simulink subsystem "Reefscape_Teleop_sub"  (R2023b)
settings: Solver=VariableStepAuto  StartTime=0.0  StopTime=10.0  RelTol=1e-3
libraries: simulink x13
settings Model: Creator=ander  LastModifiedBy=ander

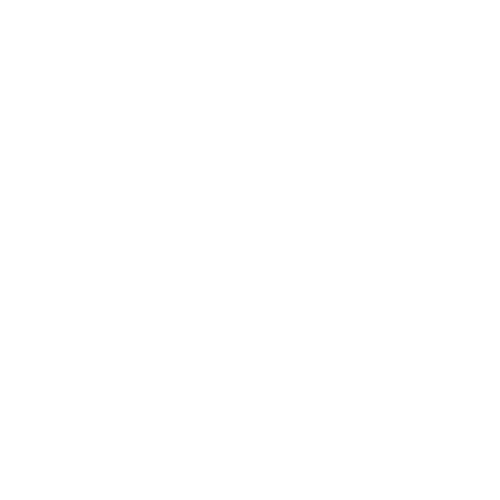
[thumbnail: Simulink's stored preview of the top-level diagram]
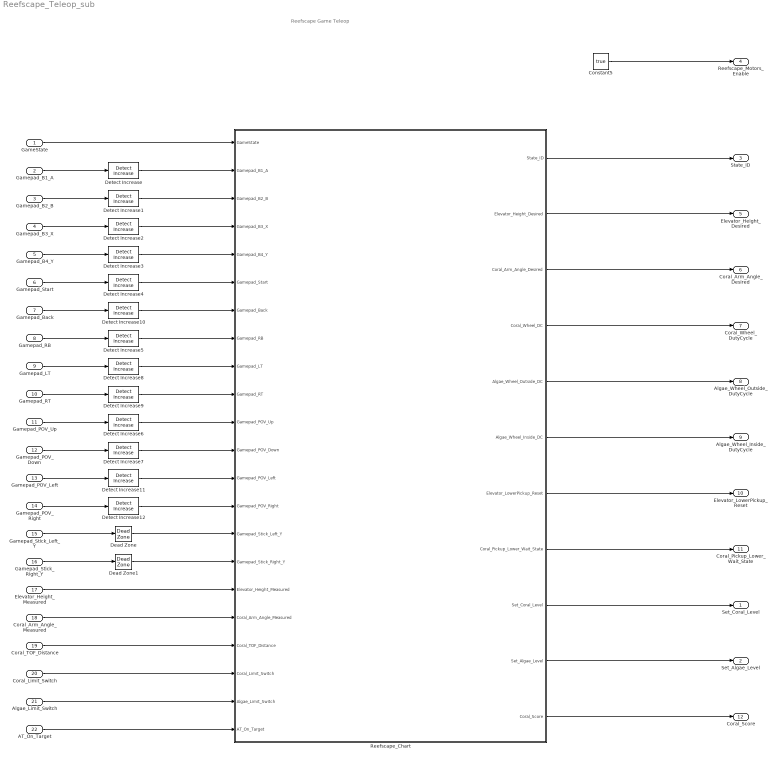
== system Reefscape_Teleop_sub ==
  note: Reefscape Game Teleop
  GameState : Inport
  Gamepad_B1_A : Inport  Port=2
  Gamepad_B2_B : Inport  Port=3
  Gamepad_B3_X : Inport  Port=4
  Gamepad_B4_Y : Inport  Port=5
  Gamepad_Start : Inport  Port=6
  Gamepad_Back : Inport  Port=7
  Gamepad_RB : Inport  Port=8
  Gamepad_LT : Inport  Port=9
  Gamepad_RT : Inport  Port=10
  Gamepad_POV_Up : Inport  Port=11
  Gamepad_POV_Down : Inport  Port=12
  Gamepad_POV_Left : Inport  Port=13
  Gamepad_POV_Right : Inport  Port=14
  Gamepad_Stick_Left_Y : Inport  Port=15
  Gamepad_Stick_Right_Y : Inport  Port=16
  Elevator_Height_Measured : Inport  Port=17
  Coral_Arm_Angle_Measured : Inport  Port=18
  Coral_TOF_Distance : Inport  Port=19
  Coral_Limit_Switch : Inport  Port=20
  Algae_Limit_Switch : Inport  Port=21
  AT_On_Target : Inport  Port=22
  Constant5 : Constant  Value=true
  Dead Zone : DeadZone  LowerValue=-0.1  UpperValue=0.1
  Dead Zone1 : DeadZone  LowerValue=-0.1  UpperValue=0.1
  Detect Increase{,1..12} (13 alike) : simulink/Logic and Bit Operations/Detect Increase  vinit=0.0  OutDataTypeStr=boolean
  Reefscape_Chart : Stateflow chart  TreatAsAtomicUnit=on
  Set_Coral_Level : Outport
  Set_Algae_Level : Outport  Port=2
  State_ID : Outport  Port=3
  Reefscape_Motors_Enable : Outport  Port=4
  Elevator_Height_Desired : Outport  Port=5
  Coral_Arm_Angle_Desired : Outport  Port=6
  Coral_Wheel_DutyCycle : Outport  Port=7
  Algae_Wheel_Outside_DutyCycle : Outport  Port=8
  Algae_Wheel_Inside_DutyCycle : Outport  Port=9
  Elevator_LowerPickup_Reset : Outport  Port=10
  Coral_Pickup_Lower_Wait_State : Outport  Port=11
  Coral_Score : Outport  Port=12
  wires:
  Reefscape_Chart/8(Coral_Pickup_Lower_Wait_State) -> Coral_Pickup_Lower_Wait_State/1
  Reefscape_Chart/5(Algae_Wheel_Outside_DC) -> Algae_Wheel_Outside_DutyCycle/1
  Detect Increase9/1 -> Reefscape_Chart/10(Gamepad_RT)
  Detect Increase8/1 -> Reefscape_Chart/9(Gamepad_LT)
  Gamepad_RT/1 -> Detect Increase9/1
  Gamepad_LT/1 -> Detect Increase8/1
  Reefscape_Chart/4(Coral_Wheel_DC) -> Coral_Wheel_DutyCycle/1
  Reefscape_Chart/3(Coral_Arm_Angle_Desired) -> Coral_Arm_Angle_Desired/1
  Reefscape_Chart/2(Elevator_Height_Desired) -> Elevator_Height_Desired/1
  Coral_Arm_Angle_Measured/1 -> Reefscape_Chart/18(Coral_Arm_Angle_Measured)
  Coral_TOF_Distance/1 -> Reefscape_Chart/19(Coral_TOF_Distance)
  Elevator_Height_Measured/1 -> Reefscape_Chart/17(Elevator_Height_Measured)
  Coral_Limit_Switch/1 -> Reefscape_Chart/20(Coral_Limit_Switch)
  Gamepad_Stick_Right_Y/1 -> Dead Zone1/1
  Gamepad_Stick_Left_Y/1 -> Dead Zone/1
  Detect Increase7/1 -> Reefscape_Chart/12(Gamepad_POV_Down)
  Detect Increase6/1 -> Reefscape_Chart/11(Gamepad_POV_Up)
  Gamepad_POV_Down/1 -> Detect Increase7/1
  Gamepad_POV_Up/1 -> Detect Increase6/1
  Detect Increase5/1 -> Reefscape_Chart/8(Gamepad_RB)
  Detect Increase4/1 -> Reefscape_Chart/6(Gamepad_Start)
  Detect Increase3/1 -> Reefscape_Chart/5(Gamepad_B4_Y)
  Detect Increase2/1 -> Reefscape_Chart/4(Gamepad_B3_X)
  Detect Increase1/1 -> Reefscape_Chart/3(Gamepad_B2_B)
  Detect Increase/1 -> Reefscape_Chart/2(Gamepad_B1_A)
  Gamepad_B1_A/1 -> Detect Increase/1
  Gamepad_B2_B/1 -> Detect Increase1/1
  Gamepad_B3_X/1 -> Detect Increase2/1
  Gamepad_B4_Y/1 -> Detect Increase3/1
  Gamepad_Start/1 -> Detect Increase4/1
  Constant5/1 -> Reefscape_Motors_Enable/1
  Gamepad_RB/1 -> Detect Increase5/1
  Algae_Limit_Switch/1 -> Reefscape_Chart/21(Algae_Limit_Switch)
  Reefscape_Chart/6(Algae_Wheel_Inside_DC) -> Algae_Wheel_Inside_DutyCycle/1
  Dead Zone/1 -> Reefscape_Chart/15(Gamepad_Stick_Left_Y)
  Dead Zone1/1 -> Reefscape_Chart/16(Gamepad_Stick_Right_Y)
  Reefscape_Chart/7(Elevator_LowerPickup_Reset) -> Elevator_LowerPickup_Reset/1
  Gamepad_Back/1 -> Detect Increase10/1
  Detect Increase10/1 -> Reefscape_Chart/7(Gamepad_Back)
  Gamepad_POV_Left/1 -> Detect Increase11/1
  Gamepad_POV_Right/1 -> Detect Increase12/1
  Detect Increase11/1 -> Reefscape_Chart/13(Gamepad_POV_Left)
  Detect Increase12/1 -> Reefscape_Chart/14(Gamepad_POV_Right)
  Reefscape_Chart/9(Set_Coral_Level) -> Set_Coral_Level/1
  Reefscape_Chart/10(Set_Algae_Level) -> Set_Algae_Level/1
  AT_On_Target/1 -> Reefscape_Chart/22(AT_On_Target)
  Reefscape_Chart/11(Coral_Score) -> Coral_Score/1
  GameState/1 -> Reefscape_Chart/1(GameState)
  Reefscape_Chart/1(State_ID) -> State_ID/1

== stateflow chart Reefscape_Teleop_sub/Reefscape_Chart ==
  state Elevator_CoralArm_CoralWheel [parallel]
    settings: executionOrder=1
    state Algae_Pickup_High
      en: State_ID = 4.3;
      Elevator_Height_Desired = Elevator_Height_Algae_High;
      Coral_Arm_Angle_Desired = Coral_Arm_Angle_Up;
      Set_Algae_Level = 3;
      du: Elevator_Height_Desired = Elevator_Height_Desired + Gamepad_Stick_Right_Y* Elevator_Height_Manual_Gain;
      Coral_Arm_Angle_Desired = Coral_Arm_Angle_Desired + Gamepad_Stick_Left_Y*Coral_Arm_Manual_Gain;
      ex: Set_Algae_Level = 0;
      state Coral_Motor_Off
        en: Coral_Wheel_DC = 0;  % off
      state Coral_Eject
        en: Coral_Wheel_DC = Coral_Motor_DC_Eject;
        timer = 0;
        du: timer = timer + 0.02;
      (default) -> Elevator_CoralArm_CoralWheel.Algae_Pickup_High.Coral_Motor_Off
      Elevator_CoralArm_CoralWheel.Algae_Pickup_High.Coral_Motor_Off -> Elevator_CoralArm_CoralWheel.Algae_Pickup_High.Coral_Eject : [Gamepad_RB]
      Elevator_CoralArm_CoralWheel.Algae_Pickup_High.Coral_Eject -> Elevator_CoralArm_CoralWheel.Algae_Pickup_High.Coral_Motor_Off : [timer >= Coral_Eject_Time]
    state Algae_Pickup_Low
      en: State_ID = 4.2;
      Elevator_Height_Desired = Elevator_Height_Algae_Low;
      Coral_Arm_Angle_Desired = Coral_Arm_Angle_Up;
      Set_Algae_Level = 2;
      du: Elevator_Height_Desired = Elevator_Height_Desired + Gamepad_Stick_Right_Y* Elevator_Height_Manual_Gain;
      Coral_Arm_Angle_Desired = Coral_Arm_Angle_Desired + Gamepad_Stick_Left_Y*Coral_Arm_Manual_Gain;
      ex: Set_Algae_Level = 0;
      state Coral_Motor_Off
        en: Coral_Wheel_DC = 0;  % off
      state Coral_Eject
        en: Coral_Wheel_DC = Coral_Motor_DC_Eject;
        timer = 0;
        du: timer = timer + 0.02;
      (default) -> Elevator_CoralArm_CoralWheel.Algae_Pickup_Low.Coral_Motor_Off
      Elevator_CoralArm_CoralWheel.Algae_Pickup_Low.Coral_Motor_Off -> Elevator_CoralArm_CoralWheel.Algae_Pickup_Low.Coral_Eject : [Gamepad_RB]
      Elevator_CoralArm_CoralWheel.Algae_Pickup_Low.Coral_Eject -> Elevator_CoralArm_CoralWheel.Algae_Pickup_Low.Coral_Motor_Off : [timer >= Coral_Eject_Time]
    state Algae_Score
      en: State_ID = 4.1;
      Elevator_Height_Desired = Elevator_Height_Algae_Score;
      Coral_Arm_Angle_Desired = Coral_Arm_Angle_Up;
      du: Elevator_Height_Desired = Elevator_Height_Desired + Gamepad_Stick_Right_Y* Elevator_Height_Manual_Gain;
      Coral_Arm_Angle_Desired = Coral_Arm_Angle_Desired + Gamepad_Stick_Left_Y*Coral_Arm_Manual_Gain;
      state Coral_Motor_Off
        en: Coral_Wheel_DC = 0;  % off
      state Coral_Eject
        en: Coral_Wheel_DC = Coral_Motor_DC_Eject;
        timer = 0;
        du: timer = timer + 0.02;
      (default) -> Elevator_CoralArm_CoralWheel.Algae_Score.Coral_Motor_Off
      Elevator_CoralArm_CoralWheel.Algae_Score.Coral_Motor_Off -> Elevator_CoralArm_CoralWheel.Algae_Score.Coral_Eject : [Gamepad_RB]
      Elevator_CoralArm_CoralWheel.Algae_Score.Coral_Eject -> Elevator_CoralArm_CoralWheel.Algae_Score.Coral_Motor_Off : [timer >= Coral_Eject_Time]
    state End_Game_Climb
      en: State_ID = 4.4;
      Elevator_Height_Desired = Elevator_Height_End_Game;
      Coral_Arm_Angle_Desired = -90;
      du: Elevator_Height_Desired = Elevator_Height_Desired + Gamepad_Stick_Right_Y* Elevator_Height_Manual_Gain;
      Coral_Arm_Angle_Desired = Coral_Arm_Angle_Desired + Gamepad_Stick_Left_Y*Coral_Arm_Manual_Gain;
      state Coral_Motor_Off
        en: Coral_Wheel_DC = 0;  % off
      state Coral_Eject
        en: Coral_Wheel_DC = Coral_Motor_DC_Eject;
        timer = 0;
        du: timer = timer + 0.02;
      (default) -> Elevator_CoralArm_CoralWheel.End_Game_Climb.Coral_Motor_Off
      Elevator_CoralArm_CoralWheel.End_Game_Climb.Coral_Motor_Off -> Elevator_CoralArm_CoralWheel.End_Game_Climb.Coral_Eject : [Gamepad_RB]
      Elevator_CoralArm_CoralWheel.End_Game_Climb.Coral_Eject -> Elevator_CoralArm_CoralWheel.End_Game_Climb.Coral_Motor_Off : [timer >= Coral_Eject_Time]
    state Elevator_Height_Bottom_pre
      en: State_ID = 0.1;
      Elevator_Height_Desired = Elevator_Height_Prepare;
      du: Elevator_Height_Desired = Elevator_Height_Desired + Gamepad_Stick_Right_Y* Elevator_Height_Manual_Gain;
      Coral_Arm_Angle_Desired = Coral_Arm_Angle_Desired + Gamepad_Stick_Left_Y*Coral_Arm_Manual_Gain;
      state Coral_Motor_Off
        en: Coral_Wheel_DC = 0;  % off
      state Coral_Eject
        en: Coral_Wheel_DC = Coral_Motor_DC_Eject;
        timer = 0;
        du: timer = timer + 0.02;
      (default) -> Elevator_CoralArm_CoralWheel.Elevator_Height_Bottom_pre.Coral_Motor_Off
      Elevator_CoralArm_CoralWheel.Elevator_Height_Bottom_pre.Coral_Motor_Off -> Elevator_CoralArm_CoralWheel.Elevator_Height_Bottom_pre.Coral_Eject : [Gamepad_RB]
      Elevator_CoralArm_CoralWheel.Elevator_Height_Bottom_pre.Coral_Eject -> Elevator_CoralArm_CoralWheel.Elevator_Height_Bottom_pre.Coral_Motor_Off : [timer >= Coral_Eject_Time]
    state Elevator_Height_Bottom
      en: State_ID = 0.2;
      Elevator_Height_Desired = Elevator_Height_Bottom;
      Coral_Arm_Angle_Desired = Coral_Arm_Angle_Up;
      du: Elevator_Height_Desired = Elevator_Height_Desired + Gamepad_Stick_Right_Y* Elevator_Height_Manual_Gain;
      Coral_Arm_Angle_Desired = Coral_Arm_Angle_Desired + Gamepad_Stick_Left_Y*Coral_Arm_Manual_Gain;
      state Coral_Motor_Off
        en: Coral_Wheel_DC = 0;  % off
      state Coral_Eject
        en: Coral_Wheel_DC = Coral_Motor_DC_Eject;
        timer = 0;
        du: timer = timer + 0.02;
      (default) -> Elevator_CoralArm_CoralWheel.Elevator_Height_Bottom.Coral_Motor_Off
      Elevator_CoralArm_CoralWheel.Elevator_Height_Bottom.Coral_Motor_Off -> Elevator_CoralArm_CoralWheel.Elevator_Height_Bottom.Coral_Eject : [Gamepad_RB]
      Elevator_CoralArm_CoralWheel.Elevator_Height_Bottom.Coral_Eject -> Elevator_CoralArm_CoralWheel.Elevator_Height_Bottom.Coral_Motor_Off : [timer >= Coral_Eject_Time]
    state Coral_Pickup
      state Set_Level [parallel]
        settings: executionOrder=2
        state None
          en: Set_L1 = false;
          Set_L2 = false;
          Set_L3 = false;
          Set_L4 = false;
        state L1
          en: Set_L1 = true;
          Set_L2 = false;
          Set_L3 = false;
          Set_L4 = false;
        state L2
          en: Set_L1 = false;
          Set_L2 = true;
          Set_L3 = false;
          Set_L4 = false;
        state L3
          en: Set_L1 = false;
          Set_L2 = false;
          Set_L3 = true;
          Set_L4 = false;
        state L4
          en: Set_L1 = false;
          Set_L2 = false;
          Set_L3 = false;
          Set_L4 = true;
        (default) -> Elevator_CoralArm_CoralWheel.Coral_Pickup.Set_Level.None
        Elevator_CoralArm_CoralWheel.Coral_Pickup.Set_Level.None -> (junction 215)
        (junction 215) -> (junction 186)
        (junction 186) -> Elevator_CoralArm_CoralWheel.Coral_Pickup.Set_Level.L1 [order 1] : [Gamepad_B1_A]
        Elevator_CoralArm_CoralWheel.Coral_Pickup.Set_Level.L1 -> (junction 200) : [Gamepad_B3_X || ...
            | Gamepad_B2_B || ...
            | Gamepad_B4_Y]
        (junction 200) -> (junction 202)
        (junction 186) -> (junction 191) [order 2]
        (junction 213) -> (junction 215)
        Elevator_CoralArm_CoralWheel.Coral_Pickup.Set_Level.L2 -> (junction 202) : [Gamepad_B1_A || ...
            | Gamepad_B2_B || ...
            | Gamepad_B4_Y]
        (junction 191) -> Elevator_CoralArm_CoralWheel.Coral_Pickup.Set_Level.L2 [order 1] : [Gamepad_B3_X]
        (junction 202) -> (junction 204)
        (junction 191) -> (junction 194) [order 2]
        (junction 194) -> Elevator_CoralArm_CoralWheel.Coral_Pickup.Set_Level.L3 [order 1] : [Gamepad_B2_B]
        Elevator_CoralArm_CoralWheel.Coral_Pickup.Set_Level.L3 -> (junction 204) : [Gamepad_B1_A || ...
            | Gamepad_B3_X || ...
            | Gamepad_B4_Y]
        (junction 194) -> (junction 197) [order 2]
        (junction 204) -> (junction 206)
        Elevator_CoralArm_CoralWheel.Coral_Pickup.Set_Level.L4 -> (junction 206) : [Gamepad_B1_A || ...
            | Gamepad_B3_X || ...
            | Gamepad_B2_B]
        (junction 197) -> Elevator_CoralArm_CoralWheel.Coral_Pickup.Set_Level.L4 : [Gamepad_B4_Y]
        (junction 206) -> (junction 211)
        (junction 211) -> (junction 213)
      state Actions [parallel]
        settings: executionOrder=1
        state Coral_Pickup_Prepare
          en: State_ID = 1.0;
          Elevator_Height_Desired = Elevator_Height_Prepare;
          Coral_Arm_Angle_Desired = -90;
          Coral_Wheel_DC = 0;  % off
          du: Elevator_Height_Desired = Elevator_Height_Desired + Gamepad_Stick_Right_Y* Elevator_Height_Manual_Gain;
          Coral_Arm_Angle_Desired = Coral_Arm_Angle_Desired + Gamepad_Stick_Left_Y*Coral_Arm_Manual_Gain;
          state Coral_Motor_Off
            en: Coral_Wheel_DC = 0;  % off
          state Coral_Eject
            en: Coral_Wheel_DC = Coral_Motor_DC_Eject;
            timer = 0;
            du: timer = timer + 0.02;
          (default) -> Elevator_CoralArm_CoralWheel.Coral_Pickup.Actions.Coral_Pickup_Prepare.Coral_Motor_Off
          Elevator_CoralArm_CoralWheel.Coral_Pickup.Actions.Coral_Pickup_Prepare.Coral_Motor_Off -> Elevator_CoralArm_CoralWheel.Coral_Pickup.Actions.Coral_Pickup_Prepare.Coral_Eject : [Gamepad_RB]
          Elevator_CoralArm_CoralWheel.Coral_Pickup.Actions.Coral_Pickup_Prepare.Coral_Eject -> Elevator_CoralArm_CoralWheel.Coral_Pickup.Actions.Coral_Pickup_Prepare.Coral_Motor_Off : [timer >= Coral_Eject_Time]
        state Coral_Pickup_Lower
          en: State_ID = 1.1;
          Elevator_Height_Desired = Elevator_Height_Lower;
          Coral_Wheel_DC = Coral_Motor_DC_Pickup;
          du: Elevator_Height_Desired = Elevator_Height_Desired + Gamepad_Stick_Right_Y* Elevator_Height_Manual_Gain;
          Coral_Arm_Angle_Desired = Coral_Arm_Angle_Desired + Gamepad_Stick_Left_Y*Coral_Arm_Manual_Gain;
        state Coral_Pickup_Lower_Wait
          en: State_ID = 1.2;
          Coral_Pickup_Lower_Wait_State = true;
          Coral_Wheel_DC = Coral_Motor_DC_Hold;
          Elevator_LowerPickup_Reset = false;
          timer = 0;
          du: timer = timer + 0.02;
          Elevator_Height_Desired = Elevator_Height_Desired + Gamepad_Stick_Right_Y* Elevator_Height_Manual_Gain;
          Coral_Arm_Angle_Desired = Coral_Arm_Angle_Desired + Gamepad_Stick_Left_Y*Coral_Arm_Manual_Gain;
          ex: Coral_Pickup_Lower_Wait_State = false;
        state Coral_Pickup_Raise
          en: State_ID = 1.3;
          Elevator_Height_Desired = Elevator_Height_Raise;
          du: Elevator_Height_Desired = Elevator_Height_Desired + Gamepad_Stick_Right_Y* Elevator_Height_Manual_Gain;
          Coral_Arm_Angle_Desired = Coral_Arm_Angle_Desired + Gamepad_Stick_Left_Y*Coral_Arm_Manual_Gain;
        Coral_Pickup_Prepare -> Coral_Pickup_Lower : [abs(Elevator_Height_Desired-Elevator_Height_Measured) <= ...
            | Elevator_Height_Error_Threshold && ...
            | abs(Coral_Arm_Angle_Desired-Coral_Arm_Angle_Measured) <= ...
            | Coral_Arm_Angle_Error_Threshold && ...
            | Coral_TOF_Distance < Coral_Detect_Distance]
        Coral_Pickup_Lower -> Coral_Pickup_Lower_Wait : [Coral_Limit_Switch]
        Coral_Pickup_Lower_Wait -> Coral_Pickup_Raise : [timer >= Elevator_LowerPickup_Time && ...
            | (Set_L1 || Set_L2 || Set_L3 || Set_L4)]
            | {Elevator_LowerPickup_Reset = true;}
    state Start
      en: State_ID = 0.0;
      Elevator_Height_Desired = Elevator_Height_Bottom;
      Coral_Arm_Angle_Desired = Coral_Arm_Angle_Up;
      Coral_Wheel_DC = 0;  % off
      state Set_Level
        state None
          en: Set_L1 = false;
          Set_L2 = false;
          Set_L3 = false;
          Set_L4 = false;
        state L1
          en: Set_L1 = true;
          Set_L2 = false;
          Set_L3 = false;
          Set_L4 = false;
        state L2
          en: Set_L1 = false;
          Set_L2 = true;
          Set_L3 = false;
          Set_L4 = false;
        state L3
          en: Set_L1 = false;
          Set_L2 = false;
          Set_L3 = true;
          Set_L4 = false;
        state L4
          en: Set_L1 = false;
          Set_L2 = false;
          Set_L3 = false;
          Set_L4 = true;
        (default) -> Elevator_CoralArm_CoralWheel.Start.Set_Level.None
        Elevator_CoralArm_CoralWheel.Start.Set_Level.None -> (junction 312)
        (junction 312) -> (junction 313)
        (junction 313) -> Elevator_CoralArm_CoralWheel.Start.Set_Level.L1 [order 1] : [Gamepad_B1_A]
        Elevator_CoralArm_CoralWheel.Start.Set_Level.L1 -> (junction 314) : [Gamepad_B3_X || ...
            | Gamepad_B2_B || ...
            | Gamepad_B4_Y]
        (junction 314) -> (junction 315)
        (junction 313) -> (junction 316) [order 2]
        (junction 321) -> (junction 312)
        Elevator_CoralArm_CoralWheel.Start.Set_Level.L2 -> (junction 315) : [Gamepad_B1_A || ...
            | Gamepad_B2_B || ...
            | Gamepad_B4_Y]
        (junction 316) -> Elevator_CoralArm_CoralWheel.Start.Set_Level.L2 [order 1] : [Gamepad_B3_X]
        (junction 315) -> (junction 318)
        (junction 316) -> (junction 317) [order 2]
        (junction 317) -> Elevator_CoralArm_CoralWheel.Start.Set_Level.L3 [order 1] : [Gamepad_B2_B]
        Elevator_CoralArm_CoralWheel.Start.Set_Level.L3 -> (junction 318) : [Gamepad_B1_A || ...
            | Gamepad_B3_X || ...
            | Gamepad_B4_Y]
        (junction 317) -> (junction 320) [order 2]
        (junction 318) -> (junction 319)
        Elevator_CoralArm_CoralWheel.Start.Set_Level.L4 -> (junction 319) : [Gamepad_B1_A || ...
            | Gamepad_B3_X || ...
            | Gamepad_B2_B]
        (junction 320) -> Elevator_CoralArm_CoralWheel.Start.Set_Level.L4 : [Gamepad_B4_Y]
        (junction 319) -> (junction 322)
        (junction 322) -> (junction 321)
      (default) -> Elevator_CoralArm_CoralWheel.Start.Set_Level
    state Start_Angle
      en: State_ID = 2.0;
      Coral_Arm_Angle_Desired = Coral_Arm_Angle_Start;
    state Coral
      ex: Set_Coral_Level = 0;
      state Coral_Score_Position
        state Level_1
          en: State_ID = 2.1;
          Set_Coral_Level = 1;
          Elevator_Height_Desired = Elevator_Height_L1;
          Coral_Arm_Angle_Desired = Coral_Arm_Angle_L1;
        state Level_2
          en: State_ID = 2.2;
          Set_Coral_Level = 2;
          Elevator_Height_Desired = Elevator_Height_L2;
          Coral_Arm_Angle_Desired = Coral_Arm_Angle_L2;
        state Level_3
          en: State_ID = 2.3;
          Set_Coral_Level = 3;
          Elevator_Height_Desired = Elevator_Height_L3;
          Coral_Arm_Angle_Desired = Coral_Arm_Angle_L3;
        state Level_4
          en: State_ID = 2.4;
          Set_Coral_Level = 4;
          Elevator_Height_Desired = Elevator_Height_L4;
          Coral_Arm_Angle_Desired = Coral_Arm_Angle_L4;
        state Manual_Adjustment
          en: State_ID = 2.5;
          Elevator_Height_Desired = Elevator_Height_Desired + Gamepad_Stick_Right_Y* Elevator_Height_Manual_Gain;
          Coral_Arm_Angle_Desired = Coral_Arm_Angle_Desired + Gamepad_Stick_Left_Y*Coral_Arm_Manual_Gain;
          du: Elevator_Height_Desired = Elevator_Height_Desired + Gamepad_Stick_Right_Y* Elevator_Height_Manual_Gain;
          Coral_Arm_Angle_Desired = Coral_Arm_Angle_Desired + Gamepad_Stick_Left_Y*Coral_Arm_Manual_Gain;
        (default) -> (junction 16)
        (junction 16) -> Level_1 [order 1] : [Set_L1 || ...
            | Gamepad_B1_A]
        (junction 16) -> (junction 19) [order 2]
        Level_1 -> (junction 120)
        (junction 120) -> (junction 122)
        (junction 19) -> Elevator_CoralArm_CoralWheel.Coral.Coral_Score_Position.Level_2 [order 1] : [Set_L2 || ...
            | Gamepad_B3_X]
        Elevator_CoralArm_CoralWheel.Coral.Coral_Score_Position.Level_2 -> (junction 122)
        (junction 19) -> (junction 22) [order 2]
        (junction 122) -> (junction 124)
        Elevator_CoralArm_CoralWheel.Coral.Coral_Score_Position.Level_3 -> (junction 124)
        (junction 22) -> Elevator_CoralArm_CoralWheel.Coral.Coral_Score_Position.Level_3 [order 1] : [Set_L3 || ...
            | Gamepad_B2_B]
        (junction 124) -> (junction 126)
        (junction 22) -> (junction 25) [order 2]
        Level_4 -> (junction 126)
        (junction 25) -> Level_4 [order 1] : [Set_L4 || ...
            | Gamepad_B4_Y]
        (junction 126) -> Elevator_CoralArm_CoralWheel.Coral.Coral_Score_Position.Manual_Adjustment : [Gamepad_Stick_Right_Y ~= 0 || ...
            | Gamepad_Stick_Left_Y ~= 0]
        (junction 25) -> Elevator_CoralArm_CoralWheel.Coral.Coral_Score_Position.Manual_Adjustment [order 2]
      state Coral_Eject
        state Level_2
          en: State_ID = 3.2;
          state Auto_Lower_Elevator
            en: Elevator_Height_Desired = Elevator_Height_Desired + Elevator_Height_Coral_Score_Lower_Rate;
            du: Elevator_Height_Desired = Elevator_Height_Desired + Elevator_Height_Coral_Score_Lower_Rate;
          state Manual_Adjustment
            en: Elevator_Height_Desired = Elevator_Height_Desired + Gamepad_Stick_Right_Y* Elevator_Height_Manual_Gain;
            Coral_Arm_Angle_Desired = Coral_Arm_Angle_Desired + Gamepad_Stick_Left_Y*Coral_Arm_Manual_Gain;
            du: Elevator_Height_Desired = Elevator_Height_Desired + Gamepad_Stick_Right_Y* Elevator_Height_Manual_Gain;
            Coral_Arm_Angle_Desired = Coral_Arm_Angle_Desired + Gamepad_Stick_Left_Y*Coral_Arm_Manual_Gain;
          (default) -> Elevator_CoralArm_CoralWheel.Coral.Coral_Eject.Level_2.Auto_Lower_Elevator
          Elevator_CoralArm_CoralWheel.Coral.Coral_Eject.Level_2.Auto_Lower_Elevator -> Elevator_CoralArm_CoralWheel.Coral.Coral_Eject.Level_2.Manual_Adjustment : [Elevator_Height_Measured <= Elevator_Height_L2_Eject]
          Elevator_CoralArm_CoralWheel.Coral.Coral_Eject.Level_2.Manual_Adjustment -> Elevator_CoralArm_CoralWheel.Coral.Coral_Eject.Level_2.Auto_Lower_Elevator : [AT_On_Target]
        state Level_3
          en: State_ID = 3.3;
          state Auto_Lower_Elevator
            en: Elevator_Height_Desired = Elevator_Height_Desired + Elevator_Height_Coral_Score_Lower_Rate;
            du: Elevator_Height_Desired = Elevator_Height_Desired + Elevator_Height_Coral_Score_Lower_Rate;
          state Manual_Adjustment
            en: Elevator_Height_Desired = Elevator_Height_Desired + Gamepad_Stick_Right_Y* Elevator_Height_Manual_Gain;
            Coral_Arm_Angle_Desired = Coral_Arm_Angle_Desired + Gamepad_Stick_Left_Y*Coral_Arm_Manual_Gain;
            du: Elevator_Height_Desired = Elevator_Height_Desired + Gamepad_Stick_Right_Y* Elevator_Height_Manual_Gain;
            Coral_Arm_Angle_Desired = Coral_Arm_Angle_Desired + Gamepad_Stick_Left_Y*Coral_Arm_Manual_Gain;
          (default) -> Elevator_CoralArm_CoralWheel.Coral.Coral_Eject.Level_3.Auto_Lower_Elevator
          Elevator_CoralArm_CoralWheel.Coral.Coral_Eject.Level_3.Auto_Lower_Elevator -> Elevator_CoralArm_CoralWheel.Coral.Coral_Eject.Level_3.Manual_Adjustment : [Elevator_Height_Measured <= Elevator_Height_L3_Eject]
          Elevator_CoralArm_CoralWheel.Coral.Coral_Eject.Level_3.Manual_Adjustment -> Elevator_CoralArm_CoralWheel.Coral.Coral_Eject.Level_3.Auto_Lower_Elevator : [AT_On_Target]
        state Level_4_Teleop
          en: State_ID = 3.4;
          state Auto_Lower_Arm
            en: Coral_Arm_Angle_Desired = Coral_Arm_Angle_Desired + Coral_Arm_Angle_Coral_Score_Lower_Rate;
            du: Coral_Arm_Angle_Desired = Coral_Arm_Angle_Desired + Coral_Arm_Angle_Coral_Score_Lower_Rate;
          state Manual_Adjustment
            en: Elevator_Height_Desired = Elevator_Height_Desired + Gamepad_Stick_Right_Y* Elevator_Height_Manual_Gain;
            Coral_Arm_Angle_Desired = Coral_Arm_Angle_Desired + Gamepad_Stick_Left_Y*Coral_Arm_Manual_Gain;
            du: Elevator_Height_Desired = Elevator_Height_Desired + Gamepad_Stick_Right_Y* Elevator_Height_Manual_Gain;
            Coral_Arm_Angle_Desired = Coral_Arm_Angle_Desired + Gamepad_Stick_Left_Y*Coral_Arm_Manual_Gain;
          (default) -> Elevator_CoralArm_CoralWheel.Coral.Coral_Eject.Level_4_Teleop.Auto_Lower_Arm
          Elevator_CoralArm_CoralWheel.Coral.Coral_Eject.Level_4_Teleop.Auto_Lower_Arm -> Elevator_CoralArm_CoralWheel.Coral.Coral_Eject.Level_4_Teleop.Manual_Adjustment : [Coral_Arm_Angle_Measured < ...
              | Coral_Arm_Angle_L4_Eject_Teleop]
          Elevator_CoralArm_CoralWheel.Coral.Coral_Eject.Level_4_Teleop.Manual_Adjustment -> Elevator_CoralArm_CoralWheel.Coral.Coral_Eject.Level_4_Teleop.Auto_Lower_Arm : [AT_On_Target]
        state Level_4_Auto
          en: State_ID = 3.5;
          state Auto_Lower_Arm
            en: Coral_Arm_Angle_Desired = Coral_Arm_Angle_Desired + Coral_Arm_Angle_Coral_Score_Lower_Rate;
            du: Coral_Arm_Angle_Desired = Coral_Arm_Angle_Desired + Coral_Arm_Angle_Coral_Score_Lower_Rate;
          state Auto_Lower_Elevator
            en: Elevator_Height_Desired = Elevator_Height_Desired + Elevator_Height_Coral_Score_Lower_Rate;
            du: Elevator_Height_Desired = Elevator_Height_Desired + Elevator_Height_Coral_Score_Lower_Rate;
          (default) -> Elevator_CoralArm_CoralWheel.Coral.Coral_Eject.Level_4_Auto.Auto_Lower_Arm
          Elevator_CoralArm_CoralWheel.Coral.Coral_Eject.Level_4_Auto.Auto_Lower_Arm -> Elevator_CoralArm_CoralWheel.Coral.Coral_Eject.Level_4_Auto.Auto_Lower_Elevator : [Coral_Arm_Angle_Measured < Coral_Arm_Angle_L4_Eject_Auto]
        state Level_4_Timer
          en: State_ID = 3.6;
          Elevator_Height_Desired = Elevator_Height_Desired + Elevator_Height_Coral_Score_Lower_Rate;
          timer = 0.02;
          du: Elevator_Height_Desired = Elevator_Height_Desired + Elevator_Height_Coral_Score_Lower_Rate;
          timer = timer + 0.02;
        state Eject
          en: State_ID = 3.7;
          Coral_Wheel_DC = Coral_Motor_DC_Eject;
          timer = 0;
          du: timer = timer + 0.02;
        state Stop
          en: State_ID = 3.8;
          Coral_Wheel_DC = 0;  % off
          Coral_Score = true;
          du: Elevator_Height_Desired = Elevator_Height_Desired + Gamepad_Stick_Right_Y* Elevator_Height_Manual_Gain;
          Coral_Arm_Angle_Desired = Coral_Arm_Angle_Desired + Gamepad_Stick_Left_Y*Coral_Arm_Manual_Gain;
          ex: Coral_Score = false;
        (default) -> (junction 268)
        (junction 268) -> Elevator_CoralArm_CoralWheel.Coral.Coral_Eject.Level_2 [order 1] : [Set_Coral_Level == 2]
        (junction 268) -> (junction 452) [order 2]
        Elevator_CoralArm_CoralWheel.Coral.Coral_Eject.Level_2 -> (junction 280) : [~Coral_Limit_Switch || ...
            | Gamepad_RB]
        (junction 280) -> (junction 456)
        (junction 452) -> Elevator_CoralArm_CoralWheel.Coral.Coral_Eject.Level_3 [order 1] : [Set_Coral_Level == 3]
        (junction 452) -> (junction 274) [order 2]
        Elevator_CoralArm_CoralWheel.Coral.Coral_Eject.Level_3 -> (junction 456) : [~Coral_Limit_Switch || ...
            | Gamepad_RB]
        (junction 456) -> (junction 279)
        (junction 274) -> Level_4_Teleop [order 1] : [Set_Coral_Level == 4 && ...
            | GameState == 2]
        Level_4_Teleop -> (junction 279) [order 1] : [Gamepad_RB]
        (junction 274) -> (junction 420) [order 2]
        (junction 279) -> (junction 496)
        Level_4_Teleop -> Level_4_Timer [order 2] : [~Coral_Limit_Switch]
        Level_4_Auto -> Level_4_Timer : [~Coral_Limit_Switch]
        (junction 420) -> Level_4_Auto [order 1] : [Set_Coral_Level == 4 && ...
            | GameState == 1]
        Level_4_Timer -> (junction 496) : [timer >= L4_Switch_Time]
        (junction 420) -> Eject [order 2] : % by default
            | % it is Set_L1
        (junction 496) -> Eject
        Eject -> Stop : [timer >= Coral_Eject_Time]
      (junction 350) -> Coral_Score_Position
      Coral_Score_Position -> Coral_Score_Position [order 1] : [Gamepad_B1_A || ...
          | Gamepad_B3_X || ...
          | Gamepad_B2_B || ...
          | Gamepad_B4_Y]
          | {Set_L1 = false;
          | Set_L2 = false;
          | Set_L3 = false;
          | Set_L4 = false;}
      Coral_Score_Position -> Elevator_CoralArm_CoralWheel.Coral.Coral_Eject [order 2] : [Gamepad_RB || ...
          | (timer_robot_target >= ...
          | AT_On_Target_Time)]
      Elevator_CoralArm_CoralWheel.Coral.Coral_Score_Position.Manual_Adjustment -> Eject : [~Coral_Limit_Switch]
    (junction 151) -> (junction 153)
    (junction 153) -> (junction 250)
    (junction 227) -> (junction 151)
    (junction 243) -> Algae_Pickup_High : [Gamepad_POV_Right]
    (junction 241) -> (junction 243) [order 2]
    Algae_Pickup_High -> (junction 227)
    (junction 228) -> (junction 227)
    (junction 241) -> Algae_Pickup_Low [order 1] : [Gamepad_POV_Left]
    (junction 239) -> (junction 241) [order 2]
    Algae_Pickup_Low -> (junction 228)
    (junction 230) -> (junction 228)
    (junction 239) -> Algae_Score [order 1] : [Gamepad_POV_Down]
    Algae_Score -> (junction 230)
    (junction 238) -> (junction 239) [order 2]
    (junction 142) -> (junction 230)
    (junction 550) -> Algae_Score
    (junction 357) -> (junction 550) [order 1] : [Algae_Limit_Switch]
    (junction 238) -> End_Game_Climb [order 1] : [Gamepad_POV_Up]
    (junction 237) -> (junction 238) [order 2]
    End_Game_Climb -> (junction 142)
    (junction 165) -> (junction 142)
    (junction 237) -> (junction 259) [order 1] : [Gamepad_Back]
    (junction 259) -> Elevator_Height_Bottom_pre [order 2]
    Elevator_Height_Bottom_pre -> (junction 165) [order 2]
    (junction 39) -> (junction 237) [order 2]
    (junction 259) -> Elevator_Height_Bottom [order 1] : [Coral_Arm_Angle_Measured >= ...
        | Coral_Arm_Angle_Start_Thresh]
    (junction 147) -> (junction 165)
    Elevator_Height_Bottom_pre -> Elevator_Height_Bottom [order 1] : [Elevator_Height_Measured > ...
        | Elevator_Height_Desired - ...
        | Elevator_Height_Error_Threshold]
    Elevator_Height_Bottom -> (junction 147)
    (junction 109) -> (junction 147)
    (junction 357) -> Elevator_Height_Bottom [order 2]
    Start -> (junction 357) [order 2] : [~Coral_Limit_Switch]
    Coral_Pickup -> (junction 109)
    Coral_Score_Position -> (junction 109) [order 3]
    (junction 250) -> (junction 39)
    (junction 39) -> Coral_Pickup_Prepare [order 1] : [Gamepad_Start && ...
        | ~Algae_Limit_Switch]
    Elevator_CoralArm_CoralWheel.Coral.Coral_Eject -> (junction 39)
    (default) -> Start
    Start -> (junction 350) [order 1] : [Coral_Limit_Switch && ...
        | Set_L1 || Set_L2 || Set_L3 || Set_L4]
    Coral_Pickup_Raise -> Start_Angle : [abs(Elevator_Height_Desired-Elevator_Height_Measured) <= ...
        | Elevator_Height_Error_Threshold && ...
        | (Set_L1 || Set_L2 || Set_L3 || Set_L4)]
    Start_Angle -> Coral_Score_Position : [Coral_Arm_Angle_Measured > Coral_Arm_Angle_Start_Thresh]
  state Algae_Wheels [parallel]
    settings: executionOrder=2
    state Algae_Pull_In
      en: Algae_Wheel_Outside_DC = Algae_Pull_In_DC;
      Algae_Wheel_Inside_DC = Algae_Pull_In_DC;
    state Algae_Hold
      en: Algae_Wheel_Outside_DC = Algae_Hold_DC;
      Algae_Wheel_Inside_DC = Algae_Hold_DC;
    state Off
      en: Algae_Wheel_Outside_DC = 0;
      Algae_Wheel_Inside_DC = 0;
    state Algae_Push_Out
      en: Algae_Wheel_Outside_DC = Algae_Push_Out_DC;
      Algae_Wheel_Inside_DC = Algae_Push_Out_DC;
      timer = 0;
      du: timer = timer + 0.02;
    Algae_Pull_In -> Algae_Hold [order 1] : [Algae_Limit_Switch]
    Off -> Algae_Pull_In [order 2] : [Gamepad_LT || ...
        | Gamepad_POV_Left || ...
        | Gamepad_POV_Right]
    Algae_Pull_In -> Algae_Push_Out [order 2] : [Gamepad_RT]
    (default) -> Off
    Off -> Algae_Hold [order 1] : [Algae_Limit_Switch]
    Algae_Push_Out -> Off : [timer >= Algae_Eject_Time]
    Off -> Algae_Push_Out [order 3] : [Gamepad_RT]
    Algae_Hold -> Algae_Push_Out : [Gamepad_RT]
  state AT_On_Target_Timer [parallel]
    settings: executionOrder=3
    state Off_Target
      en: timer_robot_target = 0;
    state On_Target
      en: timer_robot_target = 0.02;
      du: timer_robot_target = timer_robot_target + 0.02;
    (default) -> Off_Target
    Off_Target -> On_Target : [AT_On_Target]
    On_Target -> Off_Target : [~AT_On_Target]
  data: State_ID output double; GameState input uint8; Elevator_Height_Desired output double; Coral_Arm_Angle_Desired output double; Gamepad_B1_A input boolean; Gamepad_B2_B input boolean; Gamepad_B3_X input boolean; Gamepad_B4_Y input boolean; Gamepad_Start input boolean; Gamepad_Back input boolean; Gamepad_RB input boolean; Gamepad_LT input boolean; Gamepad_RT input boolean; Gamepad_POV_Up input boolean; Gamepad_POV_Down input boolean; Gamepad_POV_Left input boolean; Gamepad_POV_Right input boolean; Gamepad_Stick_Left_Y input double; Gamepad_Stick_Right_Y input double; Coral_Arm_Angle_Error_Threshold parameter double; Elevator_Height_Error_Threshold parameter double; Elevator_Height_L3 parameter double; Coral_Arm_Angle_L3 parameter double; Coral_Arm_Angle_L4 parameter double; Elevator_Height_L4 parameter double; Elevator_Height_Prepare parameter double; Elevator_Height_Lower parameter double; Elevator_Height_Raise parameter double; Elevator_Height_L1 parameter double; Coral_Arm_Angle_L1 parameter double; Elevator_Height_Bottom parameter double; Elevator_Height_L2 parameter double; Coral_Arm_Angle_L2 parameter double; Elevator_Height_Measured input double; Coral_Arm_Angle_Measured input double; Coral_TOF_Distance input double; Coral_Limit_Switch input boolean; Coral_Detect_Distance parameter double; Elevator_Height_End_Game parameter double; Coral_Arm_Manual_Gain parameter double; Coral_Eject_Time parameter double; Elevator_Height_Manual_Gain parameter double; Coral_Wheel_DC output double; timer local double; Coral_Motor_DC_Hold parameter double; Coral_Motor_DC_Eject parameter double; Coral_Motor_DC_Pickup parameter double; Algae_Limit_Switch input boolean; Algae_Wheel_Outside_DC output double; Algae_Wheel_Inside_DC output double; Algae_Pull_In_DC parameter double; Algae_Push_Out_DC parameter double; Algae_Eject_Time parameter double; Algae_Hold_DC parameter double; Elevator_LowerPickup_Time parameter double; Elevator_LowerPickup_Reset output boolean; Coral_Arm_Angle_Start_Thresh parameter double; Set_L1 local boolean; Set_L2 local boolean; Set_L3 local boolean; Set_L4 local boolean; Elevator_Height_Algae_Low parameter double; Elevator_Height_Algae_Score parameter double; Elevator_Height_Algae_High parameter double; Coral_Arm_Angle_Up parameter double; Coral_Pickup_Lower_Wait_State output boolean; Coral_Arm_Angle_Start parameter double; Set_Coral_Level output uint16; Coral_Arm_Angle_Coral_Score_Lower_Rate parameter double; Elevator_Height_Coral_Score_Lower_Rate parameter double; Coral_Arm_Angle_L4_Eject_Auto parameter double; Set_Algae_Level output uint8; AT_On_Target_Time parameter double; AT_On_Target input boolean; timer_robot_target local double; Coral_Score output boolean; Coral_Arm_Angle_L4_Eject_Teleop parameter double; Elevator_Height_L2_Eject parameter double; Elevator_Height_L3_Eject parameter double; L4_Switch_Time parameter double
